simulink model "typeAsimctrl_NB_upgrade"  (R2017b)
settings: Solver=ode45  StartTime=0.0  StopTime=12.0  RelTol=1e-3  EnableMultiTasking=on
values from neighbouring files (symbols this model uses):
  gain_actIML = 2.1e-7*1.e+6*20/(2^16)/magIM(inddc)*gain_actIML    [TypeA_reconstruction.m]
  gain_actMNL = 5.1e-6*1.e+6*20/(2^16)/magMN(inddc)*gain_actMNL    [TypeA_reconstruction.m]
  gain_actTML = 1.7e-7*1.e+6*20/(2^16)/magTM(inddc)*gain_actTML    [TypeA_reconstruction.m]
  gainBFL = 0    [main.m]
  gainIPL = 0    [main.m]
  gainSCL = 1    [TypeA_reconstruction.m]
  gainSCT = 1    [TypeA_reconstruction.m]
  sys1 = sys1_exp    [check_exportvsmake.m]    (also in sumcon2mdlconst_typeA.m = sus.ss)
undefined symbols (not defined in the file or in its folder): cMat_BF, cMat_IM, cMat_MN, cMat_TM, Filt, gain_actBFGAS, gain_actBFL, gain_actBFP, gain_actBFR, gain_actBFT, gain_actBFV, gain_actBFY, gain_actF0GAS, gain_actF1GAS, gain_actF2GAS, gain_actF3GAS, gain_actIMP, gain_actIMR, gain_actIMT, gain_actIMV, gain_actIMY, gain_actIPL, gain_actIPT, gain_actIPY, gain_actMNP, gain_actMNR, gain_actMNT, gain_actMNV, gain_actMNY, gain_actTMP, gain_actTMY, gainBFP, gainBFR, gainBFT, gainBFV, gainBFY, gainBP, gainGASBF, gainGASF0, gainGASF1, gainGASF2, gainGASF3, gainIML, gainIMP, gainIMR, gainIMT, gainIMV, gainIMY, gainIPT, gainIPY, gainLOCK_IML, gainLOCK_IMP, gainLOCK_IMY, gainMNL, gainMNLOCK_L, gainMNLOCK_P, gainMNLOCK_Y, gainMNP, gainMNR, gainMNT ... (+22)
libraries: cstblocks x77, LiveParts x77
(part 1 of 3)
settings Model: Creator=kokioktm  LastModifiedBy=ayaka
settings DataIOCC: LimitDataPoints=on  SaveFormat=Array
settings OptimizationCC: LifeSpan=inf
settings DebuggingCC: SolverPrmCheckMsg=warning  SFUnexpectedBacktrackingDiag=warning  SFNoUnconditionalDefaultTransitionDiag=warning  SFExecutionAtInitializationDiag=none
settings HardwareCC: ProdBitPerPointer=32  ProdBitPerSizeT=32  ProdBitPerPtrDiffT=32  ProdLargestAtomicFloat=None  ProdIntDivRoundTo=Undefined  ProdEndianess=Unspecified  ProdWordSize=32  ProdHWDeviceType=32-bit Generic
settings ModelReferenceCC: PropagateSignalLabelsOutOfModel=off
settings CodeAppCC: StateflowObjectComments=on
settings GRTTargetCC: TargetLangStandard=C89/C90 (ANSI)  GeneratePreprocessorConditionals=Disable all
settings ConfigComp: CovMetricSettings=dw  CovHtmlReporting=on  CovSaveCumulativeToWorkspaceVar=on  CovSaveSingleToWorkspaceVar=on  CovExternalEMLEnable=off  CovSFcnEnable=off

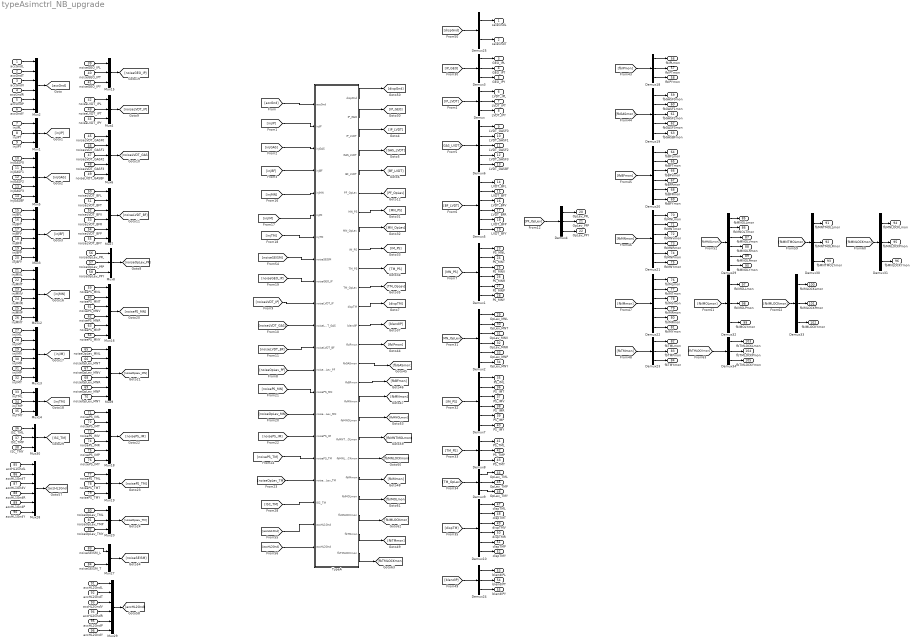
== system typeAsimctrl_NB_upgrade ==
  accGndL : Inport
  accGndT : Inport  Port=2
  accGndV : Inport  Port=3
  accGndR : Inport  Port=4
  accGndP : Inport  Port=5
  accGndY : Inport  Port=6
  injIPL : Inport  Port=7
  injIPT : Inport  Port=8
  injIPY : Inport  Port=9
  injGASF0 : Inport  Port=10
  injGASF1 : Inport  Port=11
  injGASF2 : Inport  Port=12
  injGASF3 : Inport  Port=13
  injGASBF : Inport  Port=14
  injBFL : Inport  Port=15
  injBFT : Inport  Port=16
  injBFV : Inport  Port=17
  injBFR : Inport  Port=18
  injBFP : Inport  Port=19
  injBFY : Inport  Port=20
  injMNL : Inport  Port=21
  injMNT : Inport  Port=22
  injMNV : Inport  Port=23
  injMNR : Inport  Port=24
  injMNP : Inport  Port=25
  injMNY : Inport  Port=26
  injIML : Inport  Port=27
  injIMT : Inport  Port=28
  injIMV : Inport  Port=29
  injIMR : Inport  Port=30
  injIMP : Inport  Port=31
  injIMY : Inport  Port=32
  injTML : Inport  Port=33
  injTMP : Inport  Port=34
  injTMY : Inport  Port=35
  ISC_TML : Inport  Port=36
  ISC_TMP : Inport  Port=37
  ISC_TMY : Inport  Port=38
  noiseGEO_IPL : Inport  Port=39
  noiseGEO_IPT : Inport  Port=40
  noiseGEO_IPY : Inport  Port=41
  noiseLVDT_IPL : Inport  Port=42
  noiseLVDT_IPT : Inport  Port=43
  noiseLVDT_IPY : Inport  Port=44
  noiseLVDT_GASF0 : Inport  Port=45
  noiseLVDT_GASF1 : Inport  Port=46
  noiseLVDT_GASF2 : Inport  Port=47
  noiseLVDT_GASF3 : Inport  Port=48
  noiseLVDT_GASBF : Inport  Port=49
  noiseLVDT_BFL : Inport  Port=50
  noiseLVDT_BFT : Inport  Port=51
  noiseLVDT_BFV : Inport  Port=52
  noiseLVDT_BFR : Inport  Port=53
  noiseLVDT_BFP : Inport  Port=54
  noiseLVDT_BFY : Inport  Port=55
  noiseOpLev_PFL : Inport  Port=56
  noiseOpLev_PFP : Inport  Port=57
  noiseOpLev_PFY : Inport  Port=58
  noisePS_MNL : Inport  Port=59
  noisePS_MNT : Inport  Port=60
  noisePS_MNV : Inport  Port=61
  noisePS_MNR : Inport  Port=62
  noisePS_MNP : Inport  Port=63
  noisePS_MNY : Inport  Port=64
  noiseOpLev_MNL : Inport  Port=65
  noiseOpLev_MNT : Inport  Port=66
  noiseOpLev_MNV : Inport  Port=67
  noiseOpLev_MNR : Inport  Port=68
  noiseOpLev_MNP : Inport  Port=69
  noiseOpLev_MNY : Inport  Port=70
  noisePS_IML : Inport  Port=71
  noisePS_IMT : Inport  Port=72
  noisePS_IMV : Inport  Port=73
  noisePS_IMR : Inport  Port=74
  noisePS_IMP : Inport  Port=75
  noisePS_IMY : Inport  Port=76
  noisePS_TML : Inport  Port=77
  noisePS_TMT : Inport  Port=78
  noisePS_TMY : Inport  Port=79
  noiseOpLev_TML : Inport  Port=80
  noiseOpLev_TMP : Inport  Port=81
  noiseOpLev_TMY : Inport  Port=82
  noiseSEISM_L : Inport  Port=83
  noiseSEISM_T : Inport  Port=84
  accHL1GndL : Inport  Port=85
  accHL1GndT : Inport  Port=86
  accHL1GndV : Inport  Port=87
  accHL1GndR : Inport  Port=88
  accHL1GndP : Inport  Port=89
  accHL1GndY : Inport  Port=90
  accHL2GndL : Inport  Port=91
  accHL2GndT : Inport  Port=92
  accHL2GndV : Inport  Port=93
  accHL2GndR : Inport  Port=94
  accHL2GndP : Inport  Port=95
  accHL2GndY : Inport  Port=96
  Demux{,3..4,8..9,18,23..24,30..34} (13 alike) : Demux  Outputs=3
  Demux{1..2,5,7,10,20..22,29} (9 alike) : Demux  Outputs=6
  Demux19 : Demux  Outputs=5
  Demux25 : Demux  Outputs=2
  Demux6 : Demux  Outputs=5
  Mux{1,4,8,14..15,19..20,30} (8 alike) : Mux  Inputs=3
  Mux{2..3,7,9,12..13,16,18,28..29} (10 alike) : Mux  Inputs=6
  Mux27 : Mux  Inputs=2
  Mux5 : Mux  Inputs=5
  Mux6 : Mux  Inputs=5
  TypeA : Subsystem
  seisGndL : Outport
  seisGndT : Outport  Port=2
  GEO_IPL : Outport  Port=3
  GEO_IPT : Outport  Port=4
  GEO_IPY : Outport  Port=5
  LVDT_IPL : Outport  Port=6
  LVDT_IPT : Outport  Port=7
  LVDT_IPY : Outport  Port=8
  LVDT_GASF0 : Outport  Port=9
  LVDT_GASF1 : Outport  Port=10
  LVDT_GASF2 : Outport  Port=11
  LVDT_GASF3 : Outport  Port=12
  LVDT_GASBF : Outport  Port=13
  LVDT_BFL : Outport  Port=14
  LVDT_BFT : Outport  Port=15
  LVDT_BFV : Outport  Port=16
  LVDT_BFR : Outport  Port=17
  LVDT_BFP : Outport  Port=18
  LVDT_BFY : Outport  Port=19
  OpLev_PFL : Outport  Port=20
  OpLev_PFP : Outport  Port=21
  OpLev_PFY : Outport  Port=22
  PS_MNL : Outport  Port=23
  PS_MNT : Outport  Port=24
  PS_MNV : Outport  Port=25
  PS_MNR : Outport  Port=26
  PS_MNP : Outport  Port=27
  PS_MNY : Outport  Port=28
  OpLev_MNL : Outport  Port=29
  OpLev_MNT : Outport  Port=30
  OpLev_MNV : Outport  Port=31
  OpLev_MNR : Outport  Port=32
  OpLev_MNP : Outport  Port=33
  OpLev_MNY : Outport  Port=34
  PS_IML : Outport  Port=35
  PS_IMT : Outport  Port=36
  PS_IMV : Outport  Port=37
  PS_IMR : Outport  Port=38
  PS_IMP : Outport  Port=39
  PS_IMY : Outport  Port=40
  PS_TML : Outport  Port=41
  PS_TMP : Outport  Port=42
  PS_TMY : Outport  Port=43
  OpLev_TML : Outport  Port=44
  OpLev_TMP : Outport  Port=45
  OpLev_TMY : Outport  Port=46
  dispTML : Outport  Port=47
  dispTMT : Outport  Port=48
  dispTMV : Outport  Port=49
  dispTMR : Outport  Port=50
  dispTMP : Outport  Port=51
  dispTMY : Outport  Port=52
  blendIPL : Outport  Port=53
  blendIPT : Outport  Port=54
  blendIPY : Outport  Port=55
  fbIPLmon : Outport  Port=56
  fbIPTmon : Outport  Port=57
  fbIPYmon : Outport  Port=58
  fbGASF0mon : Outport  Port=59
  fbGASF1mon : Outport  Port=60
  fbGASF2mon : Outport  Port=61
  fbGASF3mon : Outport  Port=62
  fbGASBFmon : Outport  Port=63
  fbBFLmon : Outport  Port=64
  fbBFTmon : Outport  Port=65
  fbBFVmon : Outport  Port=66
  fbBFRmon : Outport  Port=67
  fbBFPmon : Outport  Port=68
  fbBFYmon : Outport  Port=69
  fbMNLmon : Outport  Port=70
  fbMNTmon : Outport  Port=71
  fbMNVmon : Outport  Port=72
  fbMNRmon : Outport  Port=73
  fbMNPmon : Outport  Port=74
  fbMNYmon : Outport  Port=75
  fbIMLmon : Outport  Port=76
  fbIMTmon : Outport  Port=77
  fbIMVmon : Outport  Port=78
  fbIMRmon : Outport  Port=79
  fbIMPmon : Outport  Port=80
  fbIMYmon : Outport  Port=81
  fbTMLmon : Outport  Port=82
  fbTMPmon : Outport  Port=83
  fbTMYmon : Outport  Port=84
  fbMNOLLmon : Outport  Port=85
  fbMNOLTmon : Outport  Port=86
  fbMNOLVmon : Outport  Port=87
  fbMNOLRmon : Outport  Port=88
  fbMNOLPmon : Outport  Port=89
  fbMNOLYmon : Outport  Port=90
  fbMNTMOLLmon : Outport  Port=91
  fbMNTMOLPmon : Outport  Port=92
  fbMNTMOLYmon : Outport  Port=93
  fbMNLOCKLmon : Outport  Port=94
  fbMNLOCKPmon : Outport  Port=95
  fbMNLOCKYmon : Outport  Port=96
  fbIMOLLmon : Outport  Port=97
  fbIMOLPmon : Outport  Port=98
  fbIMOLYmon : Outport  Port=99
  fbIMLOCKLmon : Outport  Port=100
  fbIMLOCKPmon : Outport  Port=101
  fbIMLOCKYmon : Outport  Port=102
  fbTMLOCKLmon : Outport  Port=103
  fbTMLOCKPmon : Outport  Port=104
  fbTMLOCKYmon : Outport  Port=105
  wires:
  [accGnd] -> TypeA/1(accGnd)
  accGndT/1 -> Mux2/2
  accGndL/1 -> Mux2/1
  accGndV/1 -> Mux2/3
  accGndR/1 -> Mux2/4
  accGndP/1 -> Mux2/5
  accGndY/1 -> Mux2/6
  Mux2/1 -> [accGnd]
  injIPL/1 -> Mux1/1
  injIPT/1 -> Mux1/2
  injIPY/1 -> Mux1/3
  Mux1/1 -> [injIP]
  [injIP] -> TypeA/2(injIP)
  injGASF0/1 -> Mux5/1
  injGASF1/1 -> Mux5/2
  injGASF2/1 -> Mux5/3
  injGASF3/1 -> Mux5/4
  injGASBF/1 -> Mux5/5
  Mux5/1 -> [injGAS]
  [injGAS] -> TypeA/3(injGAS)
  injBFT/1 -> Mux3/2
  injBFL/1 -> Mux3/1
  injBFV/1 -> Mux3/3
  injBFR/1 -> Mux3/4
  injBFP/1 -> Mux3/5
  injBFY/1 -> Mux3/6
  Mux3/1 -> [injBF]
  [injBF] -> TypeA/4(injBF)
  TypeA/3(IP_LVDT) -> [IP_LVDT]
  TypeA/4(GAS_LVDT) -> [GAS_LVDT]
  TypeA/5(BF_LVDT) -> [BF_LVDT]
  TypeA/12(dispTM) -> [dispTM]
  [IP_LVDT] -> Demux/1
  Demux/1 -> LVDT_IPL/1
  Demux/2 -> LVDT_IPT/1
  Demux/3 -> LVDT_IPY/1
  [GAS_LVDT] -> Demux6/1
  Demux6/1 -> LVDT_GASF0/1
  Demux6/2 -> LVDT_GASF1/1
  Demux6/3 -> LVDT_GASF2/1
  Demux6/4 -> LVDT_GASF3/1
  Demux6/5 -> LVDT_GASBF/1
  [BF_LVDT] -> Demux5/1
  Demux5/1 -> LVDT_BFL/1
  Demux5/2 -> LVDT_BFT/1
  Demux5/3 -> LVDT_BFV/1
  Demux5/4 -> LVDT_BFR/1
  Demux5/5 -> LVDT_BFP/1
  Demux5/6 -> LVDT_BFY/1
  Demux1/1 -> PS_MNL/1
  Demux1/2 -> PS_MNT/1
  Demux1/3 -> PS_MNV/1
  Demux1/4 -> PS_MNR/1
  Demux1/5 -> PS_MNP/1
  Demux1/6 -> PS_MNY/1
  [MN_PS] -> Demux1/1
  noiseLVDT_IPL/1 -> Mux4/1
  noiseLVDT_IPT/1 -> Mux4/2
  noiseLVDT_IPY/1 -> Mux4/3
  Mux4/1 -> [noiseLVDT_IP]
  noiseLVDT_GASF0/1 -> Mux6/1
  noiseLVDT_GASF1/1 -> Mux6/2
  noiseLVDT_GASF2/1 -> Mux6/3
  noiseLVDT_GASF3/1 -> Mux6/4
  noiseLVDT_GASBF/1 -> Mux6/5
  Mux6/1 -> [noiseLVDT_GAS]
  noiseLVDT_BFT/1 -> Mux7/2
  noiseLVDT_BFL/1 -> Mux7/1
  noiseLVDT_BFV/1 -> Mux7/3
  noiseLVDT_BFR/1 -> Mux7/4
  noiseLVDT_BFP/1 -> Mux7/5
  noiseLVDT_BFY/1 -> Mux7/6
  Mux7/1 -> [noiseLVDT_BF]
  [noiseLVDT_IP] -> TypeA/10(noiseLVDT_IP)
  [noiseLVDT_GAS] -> TypeA/11(noiseLVDT_GAS)
  [noiseLVDT_BF] -> TypeA/12(noiseLVDT_BF)
  [injMN] -> TypeA/5(injMN)
  [injTM] -> TypeA/7(injTM)
  [injIM] -> TypeA/6(injIM)
  injMNT/1 -> Mux12/2
  injMNL/1 -> Mux12/1
  injMNV/1 -> Mux12/3
  injMNR/1 -> Mux12/4
  injMNP/1 -> Mux12/5
  injMNY/1 -> Mux12/6
  Mux12/1 -> [injMN]
  injIMT/1 -> Mux13/2
  injIML/1 -> Mux13/1
  injIMV/1 -> Mux13/3
  injIMR/1 -> Mux13/4
  injIMP/1 -> Mux13/5
  injIMY/1 -> Mux13/6
  Mux13/1 -> [injIM]
  injTML/1 -> Mux14/1
  injTMP/1 -> Mux14/2
  injTMY/1 -> Mux14/3
  Mux14/1 -> [injTM]
  noiseGEO_IPL/1 -> Mux15/1
  noiseGEO_IPT/1 -> Mux15/2
  noiseGEO_IPY/1 -> Mux15/3
  Mux15/1 -> [noiseGEO_IP]
  [noiseGEO_IP] -> TypeA/9(noiseGEO_IP)
  noisePS_MNT/1 -> Mux16/2
  noisePS_MNL/1 -> Mux16/1
  noisePS_MNV/1 -> Mux16/3
  noisePS_MNR/1 -> Mux16/4
  noisePS_MNP/1 -> Mux16/5
  noisePS_MNY/1 -> Mux16/6
  Mux16/1 -> [noisePS_MN]
  noiseOpLev_MNR/1 -> Mux9/4
  noiseOpLev_MNP/1 -> Mux9/5
  Mux9/1 -> [noiseOpLev_MN]
  noiseOpLev_MNY/1 -> Mux9/6
  noisePS_IMT/1 -> Mux18/2
  noisePS_IML/1 -> Mux18/1
  noisePS_IMV/1 -> Mux18/3
  noisePS_IMR/1 -> Mux18/4
  noisePS_IMP/1 -> Mux18/5
  noisePS_IMY/1 -> Mux18/6
  Mux18/1 -> [noisePS_IM]
  noisePS_TML/1 -> Mux19/1
  noisePS_TMT/1 -> Mux19/2
  Mux19/1 -> [noisePS_TM]
  noisePS_TMY/1 -> Mux19/3
  noiseOpLev_TMP/1 -> Mux20/2
  noiseOpLev_TMY/1 -> Mux20/3
  Mux20/1 -> [noiseOpLev_TM]
  [noisePS_MN] -> TypeA/14(noisePS_MN)
  [noisePS_IM] -> TypeA/16(noisePS_IM)
  [noiseOpLev_MN] -> TypeA/15(noiseOpLev_MN)
  [noisePS_TM] -> TypeA/17(noisePS_TM)
  [noiseOpLev_TM] -> TypeA/18(noiseOpLev_TM)
  [ISC_TM] -> TypeA/19(ISC_TM)
  [IP_GEO] -> Demux3/1
  Demux3/1 -> GEO_IPL/1
  Demux3/2 -> GEO_IPT/1
  Demux3/3 -> GEO_IPY/1
  TypeA/2(IP_GEO) -> [IP_GEO]
  TypeA/9(IM_PS) -> [IM_PS]
  TypeA/10(TM_PS) -> [TM_PS]
  TypeA/8(MN_OpLev) -> [MN_OpLev]
  TypeA/7(MN_PS) -> [MN_PS]
  TypeA/11(TM_OpLev) -> [TM_OpLev]
  TypeA/15(fbGASmon) -> [fbGASmon]
  TypeA/14(fbIPmon) -> [fbIPmon]
  TypeA/24(fbTMmon) -> [fbTMmon]
  TypeA/17(fbMNmon) -> [fbMNmon]
  TypeA/13(blendIP) -> [blendIP]
  TypeA/21(fbIMmon) -> [fbIMmon]
  TypeA/16(fbBFmon) -> [fbBFmon]
  [MN_OpLev] -> Demux2/1
  Demux2/5 -> OpLev_MNP/1
  Demux2/6 -> OpLev_MNY/1
  Demux2/4 -> OpLev_MNR/1
  Demux7/1 -> PS_IML/1
  Demux7/2 -> PS_IMT/1
  Demux7/3 -> PS_IMV/1
  Demux7/4 -> PS_IMR/1
  Demux7/5 -> PS_IMP/1
  Demux7/6 -> PS_IMY/1
  [IM_PS] -> Demux7/1
  Demux8/1 -> PS_TML/1
  [TM_PS] -> Demux8/1
  Demux8/2 -> PS_TMP/1
  Demux8/3 -> PS_TMY/1
  [TM_OpLev] -> Demux9/1
  Demux10/1 -> dispTML/1
  Demux10/2 -> dispTMT/1
  Demux10/3 -> dispTMV/1
  Demux10/4 -> dispTMR/1
  Demux10/5 -> dispTMP/1
  Demux10/6 -> dispTMY/1
  [dispTM] -> Demux10/1
  [fbIPmon] -> Demux18/1
  Demux18/1 -> fbIPLmon/1
  Demux18/2 -> fbIPTmon/1
  Demux18/3 -> fbIPYmon/1
  [fbGASmon] -> Demux19/1
  Demux19/1 -> fbGASF0mon/1
  Demux19/2 -> fbGASF1mon/1
  Demux19/3 -> fbGASF2mon/1
  Demux19/4 -> fbGASF3mon/1
  Demux19/5 -> fbGASBFmon/1
  [fbBFmon] -> Demux20/1
  Demux20/1 -> fbBFLmon/1
  Demux20/2 -> fbBFTmon/1
  Demux20/3 -> fbBFVmon/1
  Demux20/4 -> fbBFRmon/1
  Demux20/5 -> fbBFPmon/1
  Demux20/6 -> fbBFYmon/1
  [fbMNmon] -> Demux21/1
  Demux21/1 -> fbMNLmon/1
  Demux21/2 -> fbMNTmon/1
  Demux21/3 -> fbMNVmon/1
  Demux21/4 -> fbMNRmon/1
  Demux21/5 -> fbMNPmon/1
  Demux21/6 -> fbMNYmon/1
  [fbIMmon] -> Demux22/1
  Demux22/1 -> fbIMLmon/1
  Demux22/2 -> fbIMTmon/1
  Demux22/3 -> fbIMVmon/1
  Demux22/4 -> fbIMRmon/1
  Demux22/5 -> fbIMPmon/1
  Demux22/6 -> fbIMYmon/1
  [fbTMmon] -> Demux23/1
  Demux23/2 -> fbTMPmon/1
  Demux23/3 -> fbTMYmon/1
  Demux23/1 -> fbTMLmon/1
  Demux24/1 -> blendIPL/1
  [blendIP] -> Demux24/1
  Demux24/2 -> blendIPT/1
  Demux24/3 -> blendIPY/1
  [dispGnd] -> Demux25/1
  Demux25/1 -> seisGndL/1
  Demux25/2 -> seisGndT/1
  TypeA/1(dispGnd) -> [dispGnd]
  noiseOpLev_TML/1 -> Mux20/1
  [noiseSEISM] -> TypeA/8(noiseSEISM)
  noiseSEISM_T/1 -> Mux27/2
  Mux27/1 -> [noiseSEISM]
  noiseSEISM_L/1 -> Mux27/1
  [accHL1Gnd] -> TypeA/20(accHL1Gnd)
  [accHL2Gnd] -> TypeA/21(accHL2Gnd)
  accHL1GndT/1 -> Mux28/2
  accHL1GndL/1 -> Mux28/1
  accHL1GndV/1 -> Mux28/3
  accHL1GndR/1 -> Mux28/4
  accHL1GndP/1 -> Mux28/5
  accHL1GndY/1 -> Mux28/6
  Mux28/1 -> [accHL1Gnd]
  accHL2GndT/1 -> Mux29/2
  accHL2GndL/1 -> Mux29/1
  accHL2GndV/1 -> Mux29/3
  accHL2GndR/1 -> Mux29/4
  accHL2GndP/1 -> Mux29/5
  accHL2GndY/1 -> Mux29/6
  Mux29/1 -> [accHL2Gnd]
  TypeA/20(fbMNLOCKmon) -> [fbMNLOCKmon]
  TypeA/19(fbMNTMOLmon) -> [fbMNTMOLmon]
  TypeA/18(fbMNOLmon) -> [fbMNOLmon]
  TypeA/22(fbIMOLmon) -> [fbIMOLmon]
  TypeA/23(fbIMLOCKmon) -> [fbIMLOCKmon]
  TypeA/25(fbTMLOCKmon) -> [fbTMLOCKmon]
  [fbMNOLmon] -> Demux29/1
  [fbMNTMOLmon] -> Demux30/1
  Demux30/1 -> fbMNTMOLLmon/1
  Demux30/2 -> fbMNTMOLPmon/1
  Demux30/3 -> fbMNTMOLYmon/1
  [fbMNLOCKmon] -> Demux31/1
  Demux31/1 -> fbMNLOCKLmon/1
  Demux31/2 -> fbMNLOCKPmon/1
  Demux31/3 -> fbMNLOCKYmon/1
  [fbIMOLmon] -> Demux32/1
  Demux32/1 -> fbIMOLLmon/1
  Demux32/2 -> fbIMOLPmon/1
  Demux32/3 -> fbIMOLYmon/1
  [fbIMLOCKmon] -> Demux33/1
  Demux33/1 -> fbIMLOCKLmon/1
  Demux33/2 -> fbIMLOCKPmon/1
  Demux33/3 -> fbIMLOCKYmon/1
  [fbTMLOCKmon] -> Demux34/1
  Demux34/2 -> fbTMLOCKPmon/1
  Demux34/3 -> fbTMLOCKYmon/1
  Demux34/1 -> fbTMLOCKLmon/1
  Mux30/1 -> [ISC_TM]
  ISC_TML/1 -> Mux30/1
  ISC_TMP/1 -> Mux30/2
  ISC_TMY/1 -> Mux30/3
  [noiseOpLev_PF] -> TypeA/13(noiseOpLev_PF)
  noiseOpLev_PFL/1 -> Mux8/1
  noiseOpLev_PFY/1 -> Mux8/3
  Mux8/1 -> [noiseOpLev_PF]
  noiseOpLev_PFP/1 -> Mux8/2
  noiseOpLev_MNT/1 -> Mux9/2
  noiseOpLev_MNV/1 -> Mux9/3
  noiseOpLev_MNL/1 -> Mux9/1
  Demux2/3 -> OpLev_MNV/1
  Demux2/2 -> OpLev_MNT/1
  Demux2/1 -> OpLev_MNL/1
  TypeA/6(PF_OpLev) -> [PF_OpLev]
  Demux9/1 -> OpLev_TML/1
  Demux9/2 -> OpLev_TMP/1
  Demux9/3 -> OpLev_TMY/1
  Demux4/3 -> OpLev_PFY/1
  Demux4/1 -> OpLev_PFL/1
  Demux4/2 -> OpLev_PFP/1
  [PF_OpLev] -> Demux4/1
  Demux29/6 -> fbMNOLYmon/1
  Demux29/5 -> fbMNOLPmon/1
  Demux29/1 -> fbMNOLLmon/1
  Demux29/2 -> fbMNOLTmon/1
  Demux29/3 -> fbMNOLVmon/1
  Demux29/4 -> fbMNOLRmon/1

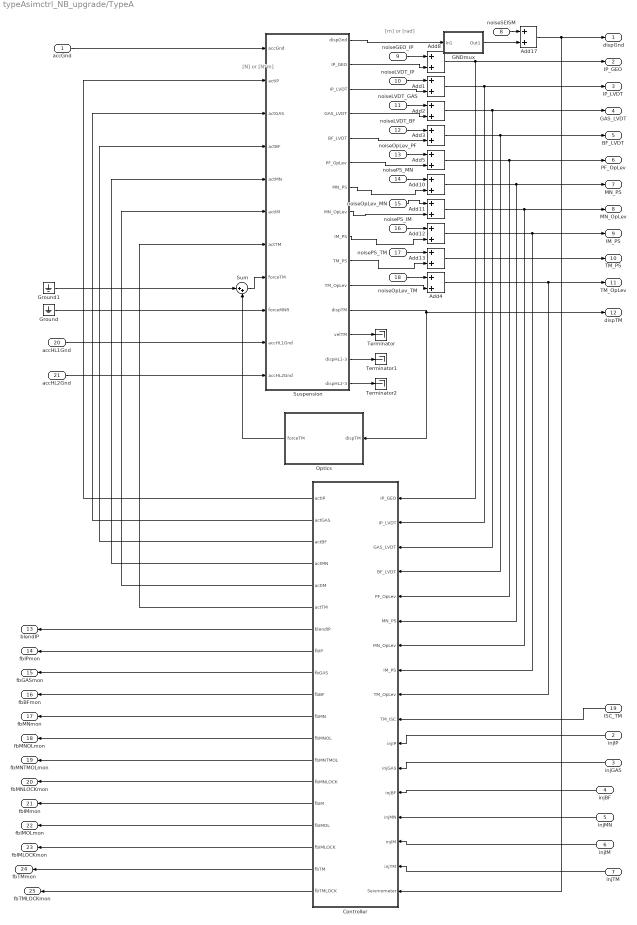
== system typeAsimctrl_NB_upgrade/TypeA ==
  note: [N] or [N*m]
  note: [m] or [rad]
  accGnd : Inport
  injIP : Inport  Port=2
  injGAS : Inport  Port=3
  injBF : Inport  Port=4
  injMN : Inport  Port=5
  injIM : Inport  Port=6
  injTM : Inport  Port=7
  noiseSEISM : Inport  Port=8
  noiseGEO_IP : Inport  Port=9
  noiseLVDT_IP : Inport  Port=10
  noiseLVDT_GAS : Inport  Port=11
  noiseLVDT_BF : Inport  Port=12
  noiseOpLev_PF : Inport  Port=13
  noisePS_MN : Inport  Port=14
  noiseOpLev_MN : Inport  Port=15
  noisePS_IM : Inport  Port=16
  noisePS_TM : Inport  Port=17
  noiseOpLev_TM : Inport  Port=18
  ISC_TM : Inport  Port=19
  accHL1Gnd : Inport  Port=20
  accHL2Gnd : Inport  Port=21
  Add{1..5,8,10..13,17} (11 alike) : Sum
  Controller : Subsystem
  GNDmux : Subsystem
  Ground : Ground
  Ground1 : Ground
  Optics : Subsystem
  Sum : Sum  Inputs=|++
  Suspension : Subsystem
  Terminator : Terminator
  Terminator1 : Terminator
  Terminator2 : Terminator
  dispGnd : Outport
  IP_GEO : Outport  Port=2
  IP_LVDT : Outport  Port=3
  GAS_LVDT : Outport  Port=4
  BF_LVDT : Outport  Port=5
  PF_OpLev : Outport  Port=6
  MN_PS : Outport  Port=7
  MN_OpLev : Outport  Port=8
  IM_PS : Outport  Port=9
  TM_PS : Outport  Port=10
  TM_OpLev : Outport  Port=11
  dispTM : Outport  Port=12
  blendIP : Outport  Port=13
  fbIPmon : Outport  Port=14
  fbGASmon : Outport  Port=15
  fbBFmon : Outport  Port=16
  fbMNmon : Outport  Port=17
  fbMNOLmon : Outport  Port=18
  fbMNTMOLmon : Outport  Port=19
  fbMNLOCKmon : Outport  Port=20
  fbIMmon : Outport  Port=21
  fbIMOLmon : Outport  Port=22
  fbIMLOCKmon : Outport  Port=23
  fbTMmon : Outport  Port=24
  fbTMLOCKmon : Outport  Port=25
  wires:
  Add1/1 -> IP_LVDT/1, Controller/2(IP_LVDT)
  Add3/1 -> Controller/4(BF_LVDT), BF_LVDT/1
  Add2/1 -> GAS_LVDT/1, Controller/3(GAS_LVDT)
  Controller/1(actIP) -> Suspension/2(actIP)
  Controller/3(actBF) -> Suspension/4(actBF)
  Add4/1 -> Controller/9(TM_OpLev), TM_OpLev/1
  accGnd/1 -> Suspension/1(accGnd)
  Controller/2(actGAS) -> Suspension/3(actGAS)
  injGAS/1 -> Controller/12(injGAS)
  injIP/1 -> Controller/11(injIP)
  injBF/1 -> Controller/13(injBF)
  Controller/10(fbBF) -> fbBFmon/1
  Controller/8(fbIP) -> fbIPmon/1
  Controller/9(fbGAS) -> fbGASmon/1
  Suspension/3(IP_LVDT) -> Add1/2
  Suspension/4(GAS_LVDT) -> Add2/2
  Suspension/5(BF_LVDT) -> Add3/2
  Suspension/11(TM_OpLev) -> Add4/2
  noiseLVDT_IP/1 -> Add1/1
  noiseLVDT_GAS/1 -> Add2/1
  noiseLVDT_BF/1 -> Add3/1
  noiseOpLev_TM/1 -> Add4/1
  Add8/1 -> Controller/1(IP_GEO), IP_GEO/1
  noiseGEO_IP/1 -> Add8/1
  Suspension/2(IP_GEO) -> Add8/2
  noisePS_MN/1 -> Add10/1
  Add10/1 -> Controller/6(MN_PS), MN_PS/1
  noiseOpLev_MN/1 -> Add11/1
  Add11/1 -> Controller/7(MN_OpLev), MN_OpLev/1
  noisePS_IM/1 -> Add12/1
  Add12/1 -> Controller/8(IM_PS), IM_PS/1
  Suspension/8(MN_OpLev) -> Add11/2
  Suspension/7(MN_PS) -> Add10/2
  Suspension/9(IM_PS) -> Add12/2
  noisePS_TM/1 -> Add13/1
  Add13/1 -> TM_PS/1
  Suspension/10(TM_PS) -> Add13/2
  injMN/1 -> Controller/14(injMN)
  injTM/1 -> Controller/16(injTM)
  injIM/1 -> Controller/15(injIM)
  Controller/4(actMN) -> Suspension/5(actMN)
  Controller/5(actIM) -> Suspension/6(actIM)
  Controller/6(actTM) -> Suspension/7(actTM)
  Controller/7(blendIP) -> blendIP/1
  Controller/18(fbTM) -> fbTMmon/1
  Controller/11(fbMN) -> fbMNmon/1
  Controller/15(fbIM) -> fbIMmon/1
  Ground/1 -> Suspension/9(forceMNR)
  noiseSEISM/1 -> Add17/1
  Add17/1 -> Controller/17(Seismometer), dispGnd/1
  Suspension/12(dispTM) -> Optics/1(dispTM), dispTM/1
  Optics/1(forceTM) -> Sum/2
  Ground1/1 -> Sum/1
  Sum/1 -> Suspension/8(forceTM)
  Suspension/1(dispGnd) -> GNDmux/1(In1)
  GNDmux/1(Out1) -> Add17/2
  accHL1Gnd/1 -> Suspension/10(accHL1Gnd)
  accHL2Gnd/1 -> Suspension/11(accHL2Gnd)
  Controller/12(fbMNOL) -> fbMNOLmon/1
  Controller/13(fbMNTMOL) -> fbMNTMOLmon/1
  Controller/14(fbMNLOCK) -> fbMNLOCKmon/1
  Controller/16(fbIMOL) -> fbIMOLmon/1
  Controller/17(fbIMLOCK) -> fbIMLOCKmon/1
  Controller/19(fbTMLOCK) -> fbTMLOCKmon/1
  Suspension/13(velTM) -> Terminator/1
  Suspension/14(dispHL1-3) -> Terminator1/1
  Suspension/15(dispHL2-3) -> Terminator2/1
  Suspension/6(PF_OpLev) -> Add5/2
  noiseOpLev_PF/1 -> Add5/1
  Add5/1 -> Controller/5(PF_OpLev), PF_OpLev/1
  ISC_TM/1 -> Controller/10(TM_ISC)

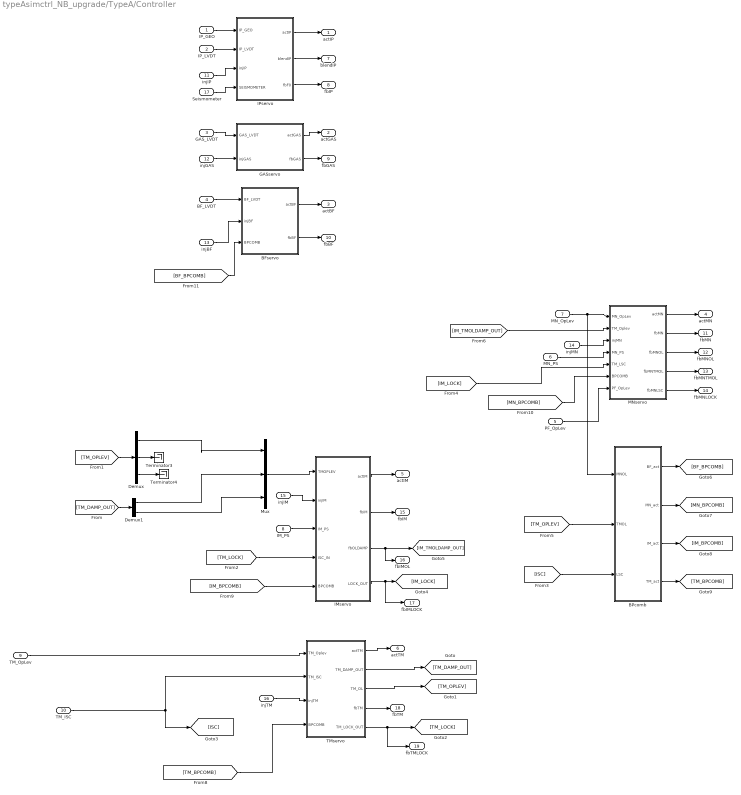
== system typeAsimctrl_NB_upgrade/TypeA/Controller ==
  IP_GEO : Inport
  IP_LVDT : Inport  Port=2
  GAS_LVDT : Inport  Port=3
  BF_LVDT : Inport  Port=4
  PF_OpLev : Inport  Port=5
  MN_PS : Inport  Port=6
  MN_OpLev : Inport  Port=7
  IM_PS : Inport  Port=8
  TM_OpLev : Inport  Port=9
  TM_ISC : Inport  Port=10
  injIP : Inport  Port=11
  injGAS : Inport  Port=12
  injBF : Inport  Port=13
  injMN : Inport  Port=14
  injIM : Inport  Port=15
  injTM : Inport  Port=16
  Seismometer : Inport  Port=17
  BFservo : Subsystem
  BPcomb : Subsystem
  Demux : Demux  Outputs=3
  Demux1 : Demux  Outputs=2
  GASservo : Subsystem
  IMservo : Subsystem
  IPservo : Subsystem
  MNservo : Subsystem
  Mux : Mux  Inputs=3
  TMservo : Subsystem
  Terminator3 : Terminator
  Terminator4 : Terminator
  actIP : Outport
  actGAS : Outport  Port=2
  actBF : Outport  Port=3
  actMN : Outport  Port=4
  actIM : Outport  Port=5
  actTM : Outport  Port=6
  blendIP : Outport  Port=7
  fbIP : Outport  Port=8
  fbGAS : Outport  Port=9
  fbBF : Outport  Port=10
  fbMN : Outport  Port=11
  fbMNOL : Outport  Port=12
  fbMNTMOL : Outport  Port=13
  fbMNLOCK : Outport  Port=14
  fbIM : Outport  Port=15
  fbIMOL : Outport  Port=16
  fbIMLOCK : Outport  Port=17
  fbTM : Outport  Port=18
  fbTMLOCK : Outport  Port=19
  wires:
  IP_LVDT/1 -> IPservo/2(IP_LVDT)
  injIP/1 -> IPservo/3(injIP)
  IPservo/3(fbF0) -> fbIP/1
  IPservo/1(actIP) -> actIP/1
  GASservo/1(actGAS) -> actGAS/1
  GASservo/2(fbGAS) -> fbGAS/1
  GAS_LVDT/1 -> GASservo/1(GAS_LVDT)
  injGAS/1 -> GASservo/2(injGAS)
  BF_LVDT/1 -> BFservo/1(BF_LVDT)
  injBF/1 -> BFservo/2(injBF)
  BFservo/1(actBF) -> actBF/1
  BFservo/2(fbBF) -> fbBF/1
  IP_GEO/1 -> IPservo/1(IP_GEO)
  IPservo/2(blendIP) -> blendIP/1
  TM_OpLev/1 -> TMservo/1(TM_Oplev)
  injTM/1 -> TMservo/3(injTM)
  MN_OpLev/1 -> BPcomb/1(MNOL), MNservo/1(MN_OpLev)
  injMN/1 -> MNservo/3(injMN)
  injIM/1 -> IMservo/2(injIM)
  TMservo/1(actTM) -> actTM/1
  TMservo/4(fbTM) -> fbTM/1
  IMservo/2(fbIM) -> fbIM/1
  IMservo/1(actIM) -> actIM/1
  MNservo/2(fbMN) -> fbMN/1
  MNservo/1(actMN) -> actMN/1
  MN_PS/1 -> MNservo/4(MN_PS)
  IM_PS/1 -> IMservo/3(IM_PS)
  TMservo/2(TM_DAMP_OUT) -> [TM_DAMP_OUT]
  [TM_OPLEV] -> Demux/1
  Demux/1 -> Mux/1
  Mux/1 -> IMservo/1(TMOPLEV)
  [TM_DAMP_OUT] -> Demux1/1
  TMservo/3(TM_OL) -> [TM_OPLEV]
  [TM_LOCK] -> IMservo/4(ISC_IN)
  IMservo/4(LOCK_OUT) -> fbIMLOCK/1, [IM_LOCK]
  [IM_LOCK] -> MNservo/5(TM_LSC)
  [IM_TMOLDAMP_OUT] -> MNservo/2(TM_Oplev)
  IMservo/3(fbOLDAMP) -> fbIMOL/1, [IM_TMOLDAMP_OUT]
  Seismometer/1 -> IPservo/4(SEISMOMETER)
  Demux1/1 -> Mux/2
  Demux1/2 -> Mux/3
  Demux/2 -> Terminator3/1
  Demux/3 -> Terminator4/1
  [ISC] -> BPcomb/3(LSC)
  [TM_OPLEV] -> BPcomb/2(TMOL)
  BPcomb/4(TM_act) -> [TM_BPCOMB]
  BPcomb/3(IM_act) -> [IM_BPCOMB]
  BPcomb/2(MN_act) -> [MN_BPCOMB]
  BPcomb/1(BF_act) -> [BF_BPCOMB]
  [TM_BPCOMB] -> TMservo/4(BPCOMB)
  [IM_BPCOMB] -> IMservo/5(BPCOMB)
  [MN_BPCOMB] -> MNservo/6(BPCOMB)
  [BF_BPCOMB] -> BFservo/3(BPCOMB)
  TMservo/5(TM_LOCK_OUT) -> fbTMLOCK/1, [TM_LOCK]
  MNservo/5(fbMNLSC) -> fbMNLOCK/1
  MNservo/3(fbMNOL) -> fbMNOL/1
  MNservo/4(fbMNTMOL) -> fbMNTMOL/1
  TM_ISC/1 -> [ISC], TMservo/2(TM_ISC)
  PF_OpLev/1 -> MNservo/7(PF_OpLev)

== system typeAsimctrl_NB_upgrade/TypeA/GNDmux ==
  In1 : Inport
  Demux : Demux
  Mux : Mux  Inputs=2
  Terminator : Terminator
  Terminator1 : Terminator
  Out1 : Outport
  wires:
  Mux/1 -> Out1/1
  Demux/4 -> Terminator/1  "Y"
  Demux/1 -> Mux/1  "L"
  Demux/3 -> Terminator1/1  "V"
  In1/1 -> Demux/1
  Demux/2 -> Mux/2  "T"

== system typeAsimctrl_NB_upgrade/TypeA/Optics ==
  dispTM : Inport
  Demux : Demux  Outputs=6
  Ground : Ground
  Kopt_angle : Gain  Gain=Kopt_angle
  Kopt_angle1 : Gain  Gain=Kopt_angle
  Kopt_len : Gain  Gain=Kopt_len
  Mux : Mux  Inputs=6
  Terminator1 : Terminator
  Terminator2 : Terminator
  Terminator3 : Terminator
  forceTM : Outport
  wires:
  dispTM/1 -> Demux/1
  Demux/6 -> Kopt_angle1/1
  Kopt_angle1/1 -> Mux/6
  Demux/5 -> Kopt_angle/1
  Kopt_angle/1 -> Mux/5
  Demux/2 -> Terminator1/1
  Demux/3 -> Terminator2/1
  Demux/4 -> Terminator3/1
  Mux/1 -> forceTM/1
  Demux/1 -> Kopt_len/1
  Kopt_len/1 -> Mux/1
  Ground/1 -> Mux/4, Mux/3, Mux/2

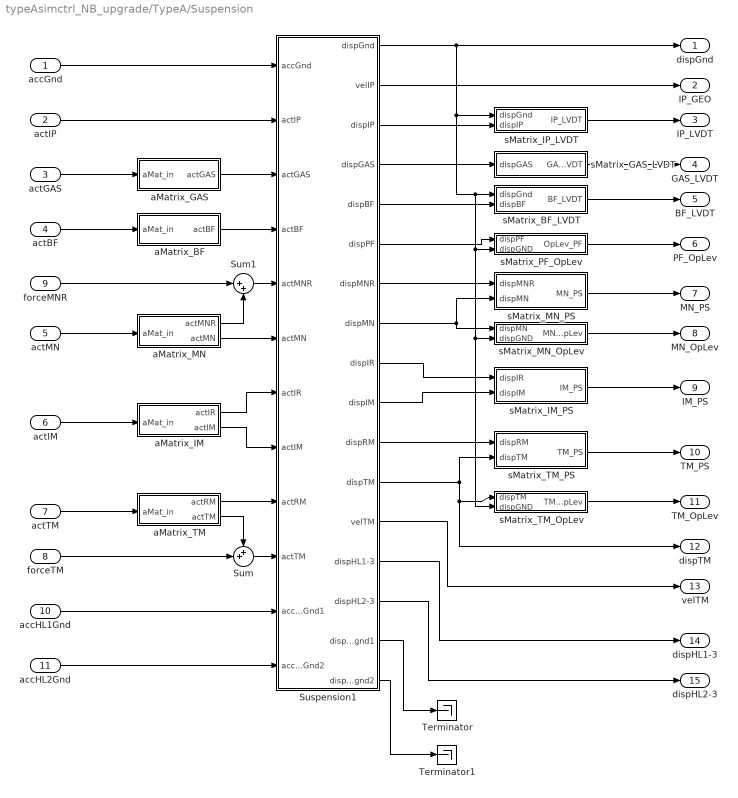
== system typeAsimctrl_NB_upgrade/TypeA/Suspension ==
  accGnd : Inport
  actIP : Inport  Port=2
  actGAS : Inport  Port=3
  actBF : Inport  Port=4
  actMN : Inport  Port=5
  actIM : Inport  Port=6
  actTM : Inport  Port=7
  forceTM : Inport  Port=8
  forceMNR : Inport  Port=9
  accHL1Gnd : Inport  Port=10
  accHL2Gnd : Inport  Port=11
  Sum : Sum  Inputs=++|
  Sum1 : Sum  Inputs=|++
  Suspension1 : Subsystem
  Terminator : Terminator
  Terminator1 : Terminator
  aMatrix_BF : Subsystem
  aMatrix_GAS : Subsystem
  aMatrix_IM : Subsystem
  aMatrix_MN : Subsystem
  aMatrix_TM : Subsystem
  sMatrix_BF_LVDT : Subsystem
  sMatrix_GAS_LVDT : Subsystem
  sMatrix_IM_PS : Subsystem
  sMatrix_IP_LVDT : Subsystem
  sMatrix_MN_OpLev : Subsystem
  sMatrix_MN_PS : Subsystem
  sMatrix_PF_OpLev : Subsystem
  sMatrix_TM_OpLev : Subsystem
  sMatrix_TM_PS : Subsystem
  dispGnd : Outport
  IP_GEO : Outport  Port=2
  IP_LVDT : Outport  Port=3
  GAS_LVDT : Outport  Port=4
  BF_LVDT : Outport  Port=5
  PF_OpLev : Outport  Port=6
  MN_PS : Outport  Port=7
  MN_OpLev : Outport  Port=8
  IM_PS : Outport  Port=9
  TM_PS : Outport  Port=10
  TM_OpLev : Outport  Port=11
  dispTM : Outport  Port=12
  velTM : Outport  Port=13
  dispHL1-3 : Outport  Port=14
  dispHL2-3 : Outport  Port=15
  wires:
  Suspension1/1(dispGnd) -> dispGnd/1, sMatrix_PF_OpLev/2(dispGND), sMatrix_MN_OpLev/2(dispGND), sMatrix_TM_OpLev/2(dispGND), sMatrix_BF_LVDT/1(dispGnd), sMatrix_IP_LVDT/1(dispGnd)
  Suspension1/3(dispIP) -> sMatrix_IP_LVDT/2(dispIP)
  Suspension1/4(dispGAS) -> sMatrix_GAS_LVDT/1(dispGAS)
  Suspension1/5(dispBF) -> sMatrix_BF_LVDT/2(dispBF)
  sMatrix_IP_LVDT/1(IP_LVDT) -> IP_LVDT/1
  sMatrix_GAS_LVDT/1(GAS_LVDT) -> GAS_LVDT/1
  sMatrix_BF_LVDT/1(BF_LVDT) -> BF_LVDT/1
  Suspension1/12(dispTM) -> dispTM/1, sMatrix_TM_OpLev/1(dispTM), sMatrix_TM_PS/2(dispTM)
  accGnd/1 -> Suspension1/1(accGnd)
  actIP/1 -> Suspension1/2(actIP)
  actGAS/1 -> aMatrix_GAS/1(aMat_in)
  actBF/1 -> aMatrix_BF/1(aMat_in)
  sMatrix_TM_OpLev/1(TM_OpLev) -> TM_OpLev/1
  aMatrix_GAS/1(actGAS) -> Suspension1/3(actGAS)
  aMatrix_BF/1(actBF) -> Suspension1/4(actBF)
  Suspension1/6(dispPF) -> sMatrix_PF_OpLev/1(dispPF)
  sMatrix_PF_OpLev/1(OpLev_PF) -> PF_OpLev/1
  Suspension1/7(dispMNR) -> sMatrix_MN_PS/1(dispMNR)
  Suspension1/8(dispMN) -> sMatrix_MN_PS/2(dispMN), sMatrix_MN_OpLev/1(dispMN)
  sMatrix_MN_PS/1(MN_PS) -> MN_PS/1
  sMatrix_MN_OpLev/1(MN_OpLev) -> MN_OpLev/1
  Suspension1/9(dispIR) -> sMatrix_IM_PS/1(dispIR)
  Suspension1/10(dispIM) -> sMatrix_IM_PS/2(dispIM)
  sMatrix_IM_PS/1(IM_PS) -> IM_PS/1
  Suspension1/11(dispRM) -> sMatrix_TM_PS/1(dispRM)
  sMatrix_TM_PS/1(TM_PS) -> TM_PS/1
  Suspension1/13(velTM) -> velTM/1
  aMatrix_MN/1(actMNR) -> Sum1/2
  aMatrix_MN/2(actMN) -> Suspension1/6(actMN)
  actMN/1 -> aMatrix_MN/1(aMat_in)
  actIM/1 -> aMatrix_IM/1(aMat_in)
  aMatrix_IM/1(actIR) -> Suspension1/7(actIR)
  aMatrix_IM/2(actIM) -> Suspension1/8(actIM)
  actTM/1 -> aMatrix_TM/1(aMat_in)
  aMatrix_TM/1(actRM) -> Suspension1/9(actRM)
  Sum/1 -> Suspension1/10(actTM)
  aMatrix_TM/2(actTM) -> Sum/1
  forceTM/1 -> Sum/2
  Suspension1/2(velIP) -> IP_GEO/1
  Sum1/1 -> Suspension1/5(actMNR)
  forceMNR/1 -> Sum1/1
  accHL1Gnd/1 -> Suspension1/11(accHLGnd1)
  accHL2Gnd/1 -> Suspension1/12(accHLGnd2)
  Suspension1/14(dispHL1-3) -> dispHL1-3/1
  Suspension1/15(dispHL2-3) -> dispHL2-3/1
  Suspension1/16(dispHLgnd1) -> Terminator/1
  Suspension1/17(dispHLgnd2) -> Terminator1/1

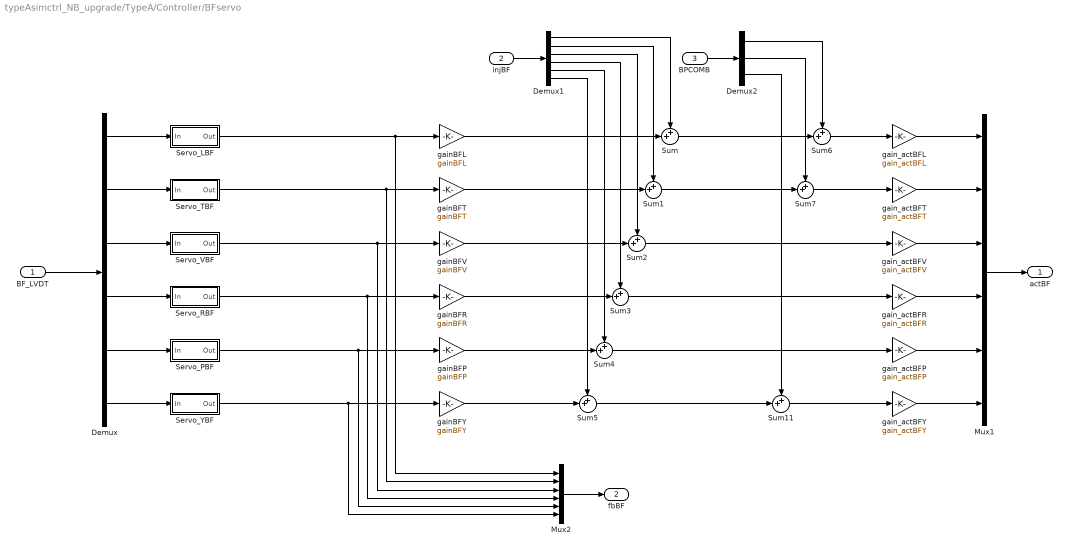
== system typeAsimctrl_NB_upgrade/TypeA/Controller/BFservo ==
  BF_LVDT : Inport
  injBF : Inport  Port=2
  BPCOMB : Inport  Port=3
  Demux : Demux  Outputs=6
  Demux1 : Demux  Outputs=6
  Demux2 : Demux  Outputs=3
  Mux1 : Mux  Inputs=6
  Mux2 : Mux  Inputs=6
  Servo_LBF : Subsystem
  Servo_PBF : Subsystem
  Servo_RBF : Subsystem
  Servo_TBF : Subsystem
  Servo_VBF : Subsystem
  Servo_YBF : Subsystem
  Sum{,1..7,11} (9 alike) : Sum  Inputs=++|
  gainBFL : Gain  Gain=gainBFL
  gainBFP : Gain  Gain=gainBFP
  gainBFR : Gain  Gain=gainBFR
  gainBFT : Gain  Gain=gainBFT
  gainBFV : Gain  Gain=gainBFV
  gainBFY : Gain  Gain=gainBFY
  gain_actBFL : Gain  Gain=gain_actBFL
  gain_actBFP : Gain  Gain=gain_actBFP
  gain_actBFR : Gain  Gain=gain_actBFR
  gain_actBFT : Gain  Gain=gain_actBFT
  gain_actBFV : Gain  Gain=gain_actBFV
  gain_actBFY : Gain  Gain=gain_actBFY
  actBF : Outport
  fbBF : Outport  Port=2
  wires:
  BF_LVDT/1 -> Demux/1
  Demux/1 -> Servo_LBF/1(In)
  Demux/2 -> Servo_TBF/1(In)
  Demux/3 -> Servo_VBF/1(In)
  Servo_LBF/1(Out) -> gainBFL/1, Mux2/1
  Servo_TBF/1(Out) -> gainBFT/1, Mux2/2
  Servo_VBF/1(Out) -> gainBFV/1, Mux2/3
  injBF/1 -> Demux1/1
  Sum2/1 -> gain_actBFV/1
  Mux1/1 -> actBF/1
  Mux2/1 -> fbBF/1
  Demux1/3 -> Sum2/1
  Demux1/2 -> Sum1/1
  Demux1/1 -> Sum/1
  Servo_RBF/1(Out) -> gainBFR/1, Mux2/4
  Servo_PBF/1(Out) -> gainBFP/1, Mux2/5
  Demux/4 -> Servo_RBF/1(In)
  Demux/5 -> Servo_PBF/1(In)
  Demux1/4 -> Sum3/1
  Demux1/5 -> Sum4/1
  Sum3/1 -> gain_actBFR/1
  Sum4/1 -> gain_actBFP/1
  Servo_YBF/1(Out) -> gainBFY/1, Mux2/6
  Demux/6 -> Servo_YBF/1(In)
  Demux1/6 -> Sum5/1
  gain_actBFV/1 -> Mux1/3
  gain_actBFY/1 -> Mux1/6
  gain_actBFR/1 -> Mux1/4
  gain_actBFT/1 -> Mux1/2
  gain_actBFL/1 -> Mux1/1
  gain_actBFP/1 -> Mux1/5
  BPCOMB/1 -> Demux2/1
  Demux2/2 -> Sum7/1
  Demux2/1 -> Sum6/1
  Demux2/3 -> Sum11/1
  Sum/1 -> Sum6/2
  Sum6/1 -> gain_actBFL/1
  Sum1/1 -> Sum7/2
  Sum7/1 -> gain_actBFT/1
  Sum5/1 -> Sum11/2
  Sum11/1 -> gain_actBFY/1
  gainBFY/1 -> Sum5/2
  gainBFR/1 -> Sum3/2
  gainBFT/1 -> Sum1/2
  gainBFV/1 -> Sum2/2
  gainBFL/1 -> Sum/2
  gainBFP/1 -> Sum4/2

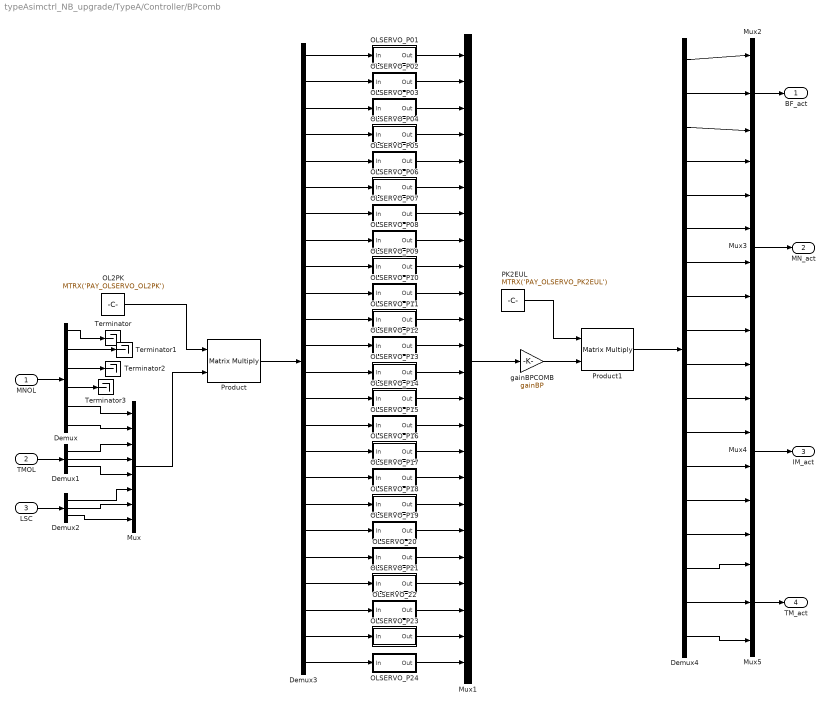
== system typeAsimctrl_NB_upgrade/TypeA/Controller/BPcomb ==
  MNOL : Inport
  TMOL : Inport  Port=2
  LSC : Inport  Port=3
  Demux : Demux  Outputs=6
  Demux1 : Demux  Outputs=3
  Demux2 : Demux  Outputs=3
  Demux3 : Demux  Outputs=24
  Demux4 : Demux  Outputs=18
  Mux : Mux  Inputs=8
  Mux1 : Mux  Inputs=24
  Mux2 : Mux  Inputs=3
  Mux3 : Mux  Inputs=6
  Mux4 : Mux  Inputs=6
  Mux5 : Mux  Inputs=3
  OL2PK : Constant  Value=MTRX('PAY_OLSERVO_OL2PK')
  OLSERVO_20 : Subsystem
  OLSERVO_22 : Subsystem
  OLSERVO_P01 : Subsystem
  OLSERVO_P02 : Subsystem
  OLSERVO_P03 : Subsystem
  OLSERVO_P04 : Subsystem
  OLSERVO_P05 : Subsystem
  OLSERVO_P06 : Subsystem
  OLSERVO_P07 : Subsystem
  OLSERVO_P08 : Subsystem
  OLSERVO_P09 : Subsystem
  OLSERVO_P10 : Subsystem
  OLSERVO_P11 : Subsystem
  OLSERVO_P12 : Subsystem
  OLSERVO_P13 : Subsystem
  OLSERVO_P14 : Subsystem
  OLSERVO_P15 : Subsystem
  OLSERVO_P16 : Subsystem
  OLSERVO_P17 : Subsystem
  OLSERVO_P18 : Subsystem
  OLSERVO_P19 : Subsystem
  OLSERVO_P21 : Subsystem
  OLSERVO_P23 : Subsystem
  OLSERVO_P24 : Subsystem
  PK2EUL : Constant  Value=MTRX('PAY_OLSERVO_PK2EUL')
  Product : Product  Multiplication=Matrix(*)
  Product1 : Product  Multiplication=Matrix(*)
  Terminator{,1..3} (4 alike) : Terminator
  gainBPCOMB : Gain  Gain=gainBP
  BF_act : Outport
  MN_act : Outport  Port=2
  IM_act : Outport  Port=3
  TM_act : Outport  Port=4
  wires:
  OL2PK/1 -> Product/1
  MNOL/1 -> Demux/1
  TMOL/1 -> Demux1/1
  LSC/1 -> Demux2/1
  Demux1/1 -> Mux/3
  Demux1/2 -> Mux/4
  Demux1/3 -> Mux/5
  Demux2/1 -> Mux/6
  Demux2/2 -> Mux/7
  Demux2/3 -> Mux/8
  Mux/1 -> Product/2
  Product/1 -> Demux3/1
  Demux3/1 -> OLSERVO_P01/1(In)
  Demux3/2 -> OLSERVO_P02/1(In)
  Demux3/3 -> OLSERVO_P03/1(In)
  Demux3/4 -> OLSERVO_P04/1(In)
  Demux3/5 -> OLSERVO_P05/1(In)
  Demux3/6 -> OLSERVO_P06/1(In)
  Demux3/7 -> OLSERVO_P07/1(In)
  Demux3/8 -> OLSERVO_P08/1(In)
  Demux3/9 -> OLSERVO_P09/1(In)
  Demux3/10 -> OLSERVO_P10/1(In)
  Demux3/11 -> OLSERVO_P11/1(In)
  Demux3/12 -> OLSERVO_P12/1(In)
  Demux3/13 -> OLSERVO_P13/1(In)
  Demux3/14 -> OLSERVO_P14/1(In)
  Demux3/15 -> OLSERVO_P15/1(In)
  Demux3/16 -> OLSERVO_P16/1(In)
  Demux3/17 -> OLSERVO_P17/1(In)
  Demux3/18 -> OLSERVO_P18/1(In)
  Demux3/19 -> OLSERVO_P19/1(In)
  Demux3/20 -> OLSERVO_20/1(In)
  Demux3/21 -> OLSERVO_P21/1(In)
  Demux3/22 -> OLSERVO_22/1(In)
  Demux3/23 -> OLSERVO_P23/1(In)
  Demux3/24 -> OLSERVO_P24/1(In)
  OLSERVO_P01/1(Out) -> Mux1/1
  OLSERVO_P02/1(Out) -> Mux1/2
  OLSERVO_P03/1(Out) -> Mux1/3
  OLSERVO_P04/1(Out) -> Mux1/4
  OLSERVO_P05/1(Out) -> Mux1/5
  OLSERVO_P06/1(Out) -> Mux1/6
  OLSERVO_P07/1(Out) -> Mux1/7
  OLSERVO_P08/1(Out) -> Mux1/8
  OLSERVO_P09/1(Out) -> Mux1/9
  OLSERVO_P10/1(Out) -> Mux1/10
  OLSERVO_P11/1(Out) -> Mux1/11
  OLSERVO_P12/1(Out) -> Mux1/12
  OLSERVO_P13/1(Out) -> Mux1/13
  OLSERVO_P14/1(Out) -> Mux1/14
  OLSERVO_P15/1(Out) -> Mux1/15
  OLSERVO_P16/1(Out) -> Mux1/16
  OLSERVO_P17/1(Out) -> Mux1/17
  OLSERVO_P18/1(Out) -> Mux1/18
  OLSERVO_P19/1(Out) -> Mux1/19
  OLSERVO_20/1(Out) -> Mux1/20
  OLSERVO_P21/1(Out) -> Mux1/21
  OLSERVO_22/1(Out) -> Mux1/22
  OLSERVO_P23/1(Out) -> Mux1/23
  OLSERVO_P24/1(Out) -> Mux1/24
  Mux1/1 -> gainBPCOMB/1
  PK2EUL/1 -> Product1/1
  Product1/1 -> Demux4/1
  Demux4/1 -> Mux2/1
  Demux4/2 -> Mux2/2
  Demux4/3 -> Mux2/3
  Mux2/1 -> BF_act/1
  Demux4/5 -> Mux3/2
  Demux4/4 -> Mux3/1
  Demux4/6 -> Mux3/3
  Demux4/7 -> Mux3/4
  Demux4/8 -> Mux3/5
  Demux4/9 -> Mux3/6
  Mux3/1 -> MN_act/1
  Demux4/11 -> Mux4/2
  Demux4/10 -> Mux4/1
  Demux4/12 -> Mux4/3
  Demux4/13 -> Mux4/4
  Demux4/14 -> Mux4/5
  Demux4/15 -> Mux4/6
  Mux4/1 -> IM_act/1
  Demux4/16 -> Mux5/1
  Demux4/17 -> Mux5/2
  Demux4/18 -> Mux5/3
  Mux5/1 -> TM_act/1
  Demux/1 -> Terminator/1
  gainBPCOMB/1 -> Product1/2
  Demux/5 -> Mux/1
  Demux/6 -> Mux/2
  Demux/2 -> Terminator1/1
  Demux/3 -> Terminator2/1
  Demux/4 -> Terminator3/1

== system typeAsimctrl_NB_upgrade/TypeA/Controller/GASservo ==
  GAS_LVDT : Inport
  injGAS : Inport  Port=2
  Demux : Demux  Outputs=5
  Demux1 : Demux  Outputs=5
  Mux1 : Mux  Inputs=5
  Mux2 : Mux  Inputs=5
  Servo_GASBF : Subsystem
  Servo_GASF0 : Subsystem
  Servo_GASF1 : Subsystem
  Servo_GASF2 : Subsystem
  Servo_GASF3 : Subsystem
  Sum{,1..4} (5 alike) : Sum  Inputs=++|
  gainGASBF : Gain  Gain=gainGASBF
  gainGASF0 : Gain  Gain=gainGASF0
  gainGASF1 : Gain  Gain=gainGASF1
  gainGASF2 : Gain  Gain=gainGASF2
  gainGASF3 : Gain  Gain=gainGASF3
  gain_actGASBF : Gain  Gain=gain_actBFGAS
  gain_actGASF0 : Gain  Gain=gain_actF0GAS
  gain_actGASF1 : Gain  Gain=gain_actF1GAS
  gain_actGASF2 : Gain  Gain=gain_actF2GAS
  gain_actGASF3 : Gain  Gain=gain_actF3GAS
  actGAS : Outport
  fbGAS : Outport  Port=2
  wires:
  GAS_LVDT/1 -> Demux/1
  Demux/1 -> Servo_GASF0/1(In)
  Demux/2 -> Servo_GASF1/1(In)
  Demux/3 -> Servo_GASF2/1(In)
  Servo_GASF0/1(Out) -> gainGASF0/1, Mux2/1
  Servo_GASF1/1(Out) -> gainGASF1/1, Mux2/2
  Servo_GASF2/1(Out) -> gainGASF2/1, Mux2/3
  injGAS/1 -> Demux1/1
  Mux1/1 -> actGAS/1
  Mux2/1 -> fbGAS/1
  Demux1/3 -> Sum2/1
  Demux1/2 -> Sum1/1
  Demux1/1 -> Sum/1
  Servo_GASF3/1(Out) -> gainGASF3/1, Mux2/4
  Servo_GASBF/1(Out) -> gainGASBF/1, Mux2/5
  Demux/4 -> Servo_GASF3/1(In)
  Demux/5 -> Servo_GASBF/1(In)
  Demux1/4 -> Sum3/1
  Demux1/5 -> Sum4/1
  gain_actGASF0/1 -> Mux1/1
  gain_actGASF2/1 -> Mux1/3
  gain_actGASF1/1 -> Mux1/2
  gain_actGASF3/1 -> Mux1/4
  gain_actGASBF/1 -> Mux1/5
  Sum/1 -> gain_actGASF0/1
  Sum2/1 -> gain_actGASF2/1
  Sum1/1 -> gain_actGASF1/1
  Sum3/1 -> gain_actGASF3/1
  Sum4/1 -> gain_actGASBF/1
  gainGASBF/1 -> Sum4/2
  gainGASF1/1 -> Sum1/2
  gainGASF2/1 -> Sum2/2
  gainGASF3/1 -> Sum3/2
  gainGASF0/1 -> Sum/2

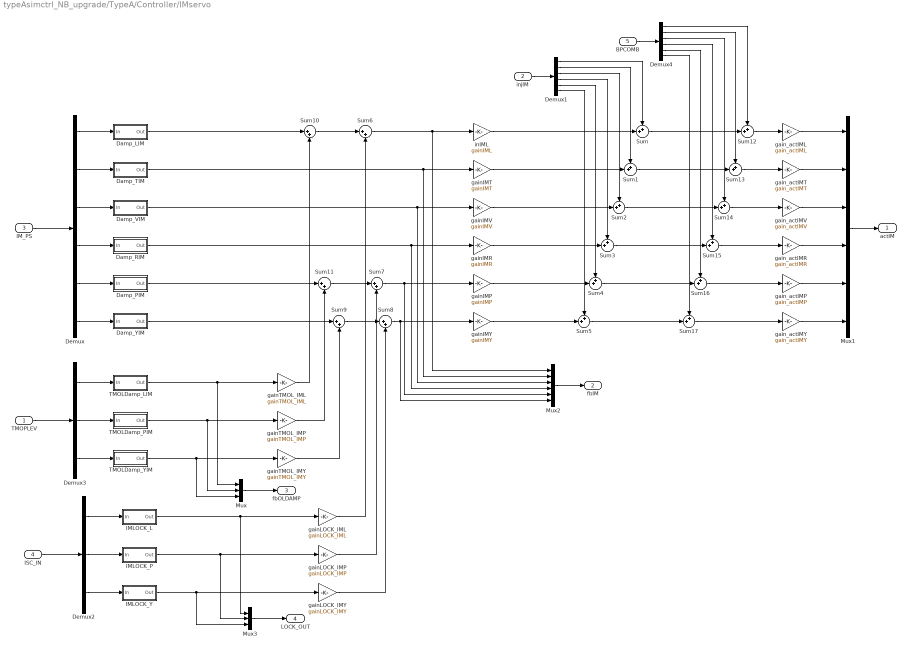
== system typeAsimctrl_NB_upgrade/TypeA/Controller/IMservo ==
  TMOPLEV : Inport
  injIM : Inport  Port=2
  IM_PS : Inport  Port=3
  ISC_IN : Inport  Port=4
  BPCOMB : Inport  Port=5
  Damp_LIM : Subsystem
  Damp_PIM : Subsystem
  Damp_RIM : Subsystem
  Damp_TIM : Subsystem
  Damp_VIM : Subsystem
  Damp_YIM : Subsystem
  Demux : Demux  Outputs=6
  Demux1 : Demux  Outputs=6
  Demux2 : Demux  Outputs=3
  Demux3 : Demux  Outputs=3
  Demux4 : Demux  Outputs=6
  IMLOCK_L : Subsystem
  IMLOCK_P : Subsystem
  IMLOCK_Y : Subsystem
  Mux : Mux  Inputs=3
  Mux1 : Mux  Inputs=6
  Mux2 : Mux  Inputs=6
  Mux3 : Mux  Inputs=3
  Sum{,1..5,12..17} (12 alike) : Sum  Inputs=++|
  Sum{6..11} (6 alike) : Sum  Inputs=|++
  TMOLDamp_LIM : Subsystem
  TMOLDamp_PIM : Subsystem
  TMOLDamp_YIM : Subsystem
  gainIMP : Gain  Gain=gainIMP
  gainIMR : Gain  Gain=gainIMR
  gainIMT : Gain  Gain=gainIMT
  gainIMV : Gain  Gain=gainIMV
  gainIMY : Gain  Gain=gainIMY
  gainLOCK_IML : Gain  Gain=gainLOCK_IML
  gainLOCK_IMP : Gain  Gain=gainLOCK_IMP
  gainLOCK_IMY : Gain  Gain=gainLOCK_IMY
  gainTMOL_IML : Gain  Gain=gainTMOL_IML
  gainTMOL_IMP : Gain  Gain=gainTMOL_IMP
  gainTMOL_IMY : Gain  Gain=gainTMOL_IMY
  gain_actIML : Gain  Gain=gain_actIML
  gain_actIMP : Gain  Gain=gain_actIMP
  gain_actIMR : Gain  Gain=gain_actIMR
  gain_actIMT : Gain  Gain=gain_actIMT
  gain_actIMV : Gain  Gain=gain_actIMV
  gain_actIMY : Gain  Gain=gain_actIMY
  inIML : Gain  Gain=gainIML
  actIM : Outport
  fbIM : Outport  Port=2
  fbOLDAMP : Outport  Port=3
  LOCK_OUT : Outport  Port=4
  wires:
  injIM/1 -> Demux1/1
  Mux1/1 -> actIM/1
  Mux2/1 -> fbIM/1
  Demux1/3 -> Sum2/1
  Demux1/2 -> Sum1/1
  Demux1/1 -> Sum/1
  Demux1/4 -> Sum3/1
  Demux1/5 -> Sum4/1
  Demux1/6 -> Sum5/1
  gain_actIMV/1 -> Mux1/3
  gain_actIMY/1 -> Mux1/6
  gain_actIMR/1 -> Mux1/4
  gain_actIMT/1 -> Mux1/2
  gain_actIML/1 -> Mux1/1
  gain_actIMP/1 -> Mux1/5
  TMOPLEV/1 -> Demux3/1
  Demux3/1 -> TMOLDamp_LIM/1(In)
  Demux3/2 -> TMOLDamp_PIM/1(In)
  Demux3/3 -> TMOLDamp_YIM/1(In)
  TMOLDamp_LIM/1(Out) -> Mux/1, gainTMOL_IML/1
  TMOLDamp_PIM/1(Out) -> Mux/2, gainTMOL_IMP/1
  TMOLDamp_YIM/1(Out) -> Mux/3, gainTMOL_IMY/1
  IM_PS/1 -> Demux/1
  Demux/1 -> Damp_LIM/1(In)
  Demux/2 -> Damp_TIM/1(In)
  Demux/3 -> Damp_VIM/1(In)
  Demux/4 -> Damp_RIM/1(In)
  Demux/5 -> Damp_PIM/1(In)
  Demux/6 -> Damp_YIM/1(In)
  Damp_LIM/1(Out) -> Sum10/1
  Damp_TIM/1(Out) -> Mux2/2, gainIMT/1
  Damp_VIM/1(Out) -> Mux2/3, gainIMV/1
  Damp_RIM/1(Out) -> Mux2/4, gainIMR/1
  Damp_PIM/1(Out) -> Sum11/1
  Damp_YIM/1(Out) -> Sum9/1
  Mux/1 -> fbOLDAMP/1
  ISC_IN/1 -> Demux2/1
  Demux2/1 -> IMLOCK_L/1(In)
  Demux2/2 -> IMLOCK_P/1(In)
  Demux2/3 -> IMLOCK_Y/1(In)
  IMLOCK_L/1(Out) -> gainLOCK_IML/1, Mux3/1
  IMLOCK_P/1(Out) -> gainLOCK_IMP/1, Mux3/2
  IMLOCK_Y/1(Out) -> gainLOCK_IMY/1, Mux3/3
  Mux3/1 -> LOCK_OUT/1
  Sum10/1 -> Sum6/1
  Sum6/1 -> Mux2/1, inIML/1
  Sum9/1 -> Sum8/1
  Sum8/1 -> Mux2/6, gainIMY/1
  Sum11/1 -> Sum7/1
  Sum7/1 -> Mux2/5, gainIMP/1
  BPCOMB/1 -> Demux4/1
  Demux4/3 -> Sum14/1
  Demux4/2 -> Sum13/1
  Demux4/1 -> Sum12/1
  Demux4/4 -> Sum15/1
  Demux4/5 -> Sum16/1
  Demux4/6 -> Sum17/1
  Sum/1 -> Sum12/2
  Sum12/1 -> gain_actIML/1
  Sum1/1 -> Sum13/2
  Sum13/1 -> gain_actIMT/1
  Sum2/1 -> Sum14/2
  Sum14/1 -> gain_actIMV/1
  Sum3/1 -> Sum15/2
  Sum15/1 -> gain_actIMR/1
  Sum4/1 -> Sum16/2
  Sum16/1 -> gain_actIMP/1
  Sum5/1 -> Sum17/2
  Sum17/1 -> gain_actIMY/1
  gainLOCK_IML/1 -> Sum6/2
  gainLOCK_IMY/1 -> Sum8/2
  gainLOCK_IMP/1 -> Sum7/2
  gainTMOL_IMY/1 -> Sum9/2
  gainTMOL_IMP/1 -> Sum11/2
  gainTMOL_IML/1 -> Sum10/2
  gainIMV/1 -> Sum2/2
  gainIMR/1 -> Sum3/2
  gainIMY/1 -> Sum5/2
  inIML/1 -> Sum/2
  gainIMT/1 -> Sum1/2
  gainIMP/1 -> Sum4/2

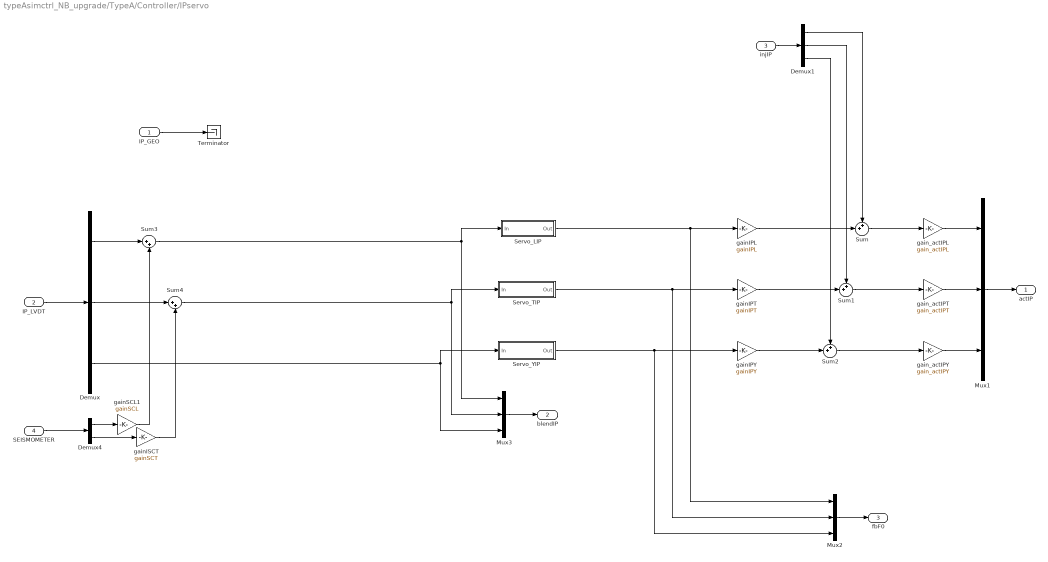
== system typeAsimctrl_NB_upgrade/TypeA/Controller/IPservo ==
  IP_GEO : Inport
  IP_LVDT : Inport  Port=2
  injIP : Inport  Port=3
  SEISMOMETER : Inport  Port=4
  Demux : Demux  Outputs=3
  Demux1 : Demux  Outputs=3
  Demux4 : Demux  Outputs=2
  Mux1 : Mux  Inputs=3
  Mux2 : Mux  Inputs=3
  Mux3 : Mux  Inputs=3
  Servo_LIP : Subsystem
  Servo_TIP : Subsystem
  Servo_YIP : Subsystem
  Sum : Sum  Inputs=++|
  Sum1 : Sum  Inputs=++|
  Sum2 : Sum  Inputs=++|
  Sum3 : Sum  Inputs=|++
  Sum4 : Sum  Inputs=|++
  Terminator : Terminator
  gainIPL : Gain  Gain=gainIPL
  gainIPT : Gain  Gain=gainIPT
  gainIPY : Gain  Gain=gainIPY
  gainISCT : Gain  Gain=gainSCT
  gainSCL1 : Gain  Gain=gainSCL
  gain_actIPL : Gain  Gain=gain_actIPL
  gain_actIPT : Gain  Gain=gain_actIPT
  gain_actIPY : Gain  Gain=gain_actIPY
  actIP : Outport
  blendIP : Outport  Port=2
  fbF0 : Outport  Port=3
  wires:
  IP_LVDT/1 -> Demux/1
  Servo_LIP/1(Out) -> Mux2/1, gainIPL/1
  Servo_TIP/1(Out) -> Mux2/2, gainIPT/1
  Servo_YIP/1(Out) -> Mux2/3, gainIPY/1
  injIP/1 -> Demux1/1
  Sum1/1 -> gain_actIPT/1
  Sum2/1 -> gain_actIPY/1
  Sum/1 -> gain_actIPL/1
  Mux1/1 -> actIP/1
  Mux2/1 -> fbF0/1
  Demux1/3 -> Sum2/1
  Demux1/2 -> Sum1/1
  Demux1/1 -> Sum/1
  gain_actIPT/1 -> Mux1/2
  gain_actIPL/1 -> Mux1/1
  gain_actIPY/1 -> Mux1/3
  IP_GEO/1 -> Terminator/1
  Sum3/1 -> Servo_LIP/1(In), Mux3/1
  Sum4/1 -> Servo_TIP/1(In), Mux3/2
  Demux/3 -> Servo_YIP/1(In), Mux3/3
  Mux3/1 -> blendIP/1
  SEISMOMETER/1 -> Demux4/1
  Demux/1 -> Sum3/1
  Demux/2 -> Sum4/1
  Demux4/1 -> gainSCL1/1
  Demux4/2 -> gainISCT/1
  gainIPL/1 -> Sum/2
  gainIPT/1 -> Sum1/2
  gainIPY/1 -> Sum2/2
  gainSCL1/1 -> Sum3/2
  gainISCT/1 -> Sum4/2

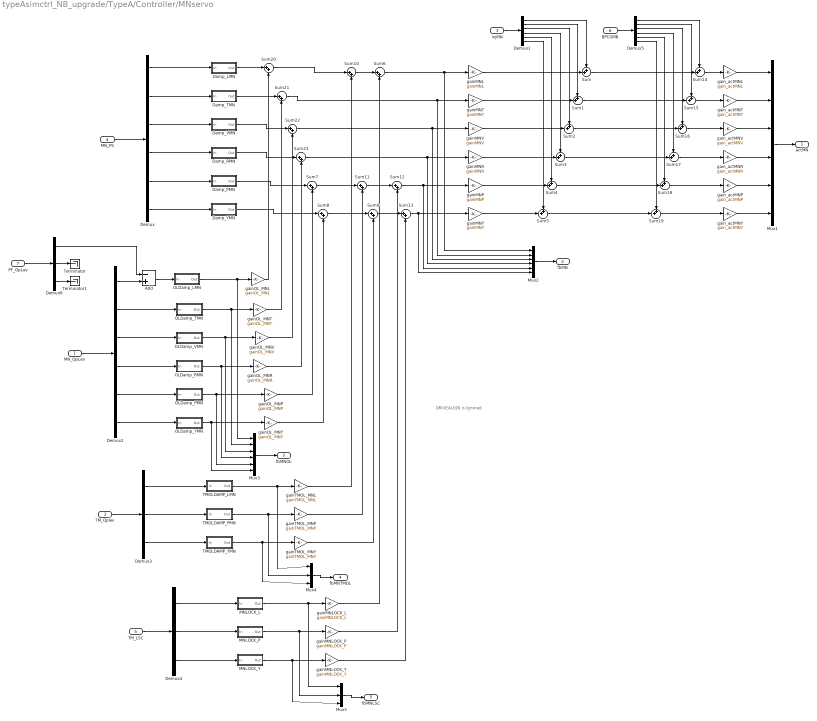
== system typeAsimctrl_NB_upgrade/TypeA/Controller/MNservo ==
  note: DRIVEALIGN is Ignored
  MN_OpLev : Inport
  TM_Oplev : Inport  Port=2
  injMN : Inport  Port=3
  MN_PS : Inport  Port=4
  TM_LSC : Inport  Port=5
  BPCOMB : Inport  Port=6
  PF_OpLev : Inport  Port=7
  Add : Sum  Inputs=-+
  Damp_LMN : Subsystem
  Damp_PMN : Subsystem
  Damp_RMN : Subsystem
  Damp_TMN : Subsystem
  Damp_VMN : Subsystem
  Damp_YMN : Subsystem
  Demux{,1..2,5} (4 alike) : Demux  Outputs=6
  Demux3 : Demux  Outputs=3
  Demux4 : Demux  Outputs=3
  Demux6 : Demux  Outputs=3
  MNLOCK_L : Subsystem
  MNLOCK_P : Subsystem
  MNLOCK_Y : Subsystem
  Mux1 : Mux  Inputs=6
  Mux2 : Mux  Inputs=6
  Mux3 : Mux  Inputs=6
  Mux4 : Mux  Inputs=3
  Mux5 : Mux  Inputs=3
  OLDamp_LMN : Subsystem
  OLDamp_PMN : Subsystem
  OLDamp_RMN : Subsystem
  OLDamp_TMN : Subsystem
  OLDamp_VMN : Subsystem
  OLDamp_YMN : Subsystem
  Sum{,1..5,14..19} (12 alike) : Sum  Inputs=++|
  Sum{6..13,20..23} (12 alike) : Sum  Inputs=|++
  TMOLDAMP_LMN : Subsystem
  TMOLDAMP_PMN : Subsystem
  TMOLDAMP_YMN : Subsystem
  Terminator : Terminator
  Terminator1 : Terminator
  gainMNL : Gain  Gain=gainMNL
  gainMNLOCK_L : Gain  Gain=gainMNLOCK_L
  gainMNLOCK_P : Gain  Gain=gainMNLOCK_P
  gainMNLOCK_Y : Gain  Gain=gainMNLOCK_Y
  gainMNP : Gain  Gain=gainMNP
  gainMNR : Gain  Gain=gainMNR
  gainMNT : Gain  Gain=gainMNT
  gainMNV : Gain  Gain=gainMNV
  gainMNY : Gain  Gain=gainMNY
  gainOL_MNL : Gain  Gain=gainOL_MNL
  gainOL_MNP : Gain  Gain=gainOL_MNP
  gainOL_MNR : Gain  Gain=gainOL_MNR
  gainOL_MNT : Gain  Gain=gainOL_MNT
  gainOL_MNV : Gain  Gain=gainOL_MNV
  gainOL_MNY : Gain  Gain=gainOL_MNY
  gainTMOL_MNL : Gain  Gain=gainTMOL_MNL
  gainTMOL_MNP : Gain  Gain=gainTMOL_MNP
  gainTMOL_MNY : Gain  Gain=gainTMOL_MNY
  gain_actMNL : Gain  Gain=gain_actMNL
  gain_actMNP : Gain  Gain=gain_actMNP
  gain_actMNR : Gain  Gain=gain_actMNR
  gain_actMNT : Gain  Gain=gain_actMNT
  gain_actMNV : Gain  Gain=gain_actMNV
  gain_actMNY : Gain  Gain=gain_actMNY
  actMN : Outport
  fbMN : Outport  Port=2
  fbMNOL : Outport  Port=3
  fbMNTMOL : Outport  Port=4
  fbMNLSC : Outport  Port=5
  wires:
  injMN/1 -> Demux1/1
  Mux1/1 -> actMN/1
  Mux2/1 -> fbMN/1
  Demux1/3 -> Sum2/1
  Demux1/2 -> Sum1/1
  Demux1/1 -> Sum/1
  Demux1/4 -> Sum3/1
  Demux1/5 -> Sum4/1
  Demux1/6 -> Sum5/1
  gain_actMNV/1 -> Mux1/3
  gain_actMNY/1 -> Mux1/6
  gain_actMNR/1 -> Mux1/4
  gain_actMNT/1 -> Mux1/2
  gain_actMNL/1 -> Mux1/1
  gain_actMNP/1 -> Mux1/5
  TMOLDAMP_YMN/1(Out) -> Mux4/3, gainTMOL_MNY/1
  OLDamp_PMN/1(Out) -> Mux3/5, gainOL_MNP/1
  OLDamp_YMN/1(Out) -> Mux3/6, gainOL_MNY/1
  MN_OpLev/1 -> Demux2/1
  TM_Oplev/1 -> Demux3/1
  Demux3/1 -> TMOLDAMP_LMN/1(In)
  gainOL_MNP/1 -> Sum7/2
  gainOL_MNY/1 -> Sum8/2
  Sum7/1 -> Sum11/1
  gainTMOL_MNL/1 -> Sum10/2
  gainTMOL_MNP/1 -> Sum11/2
  gainTMOL_MNY/1 -> Sum9/2
  Sum8/1 -> Sum9/1
  Demux3/2 -> TMOLDAMP_PMN/1(In)
  Demux3/3 -> TMOLDAMP_YMN/1(In)
  Sum21/1 -> Mux2/2, gainMNT/1
  Sum22/1 -> Mux2/3, gainMNV/1
  Sum23/1 -> Mux2/4, gainMNR/1
  MN_PS/1 -> Demux/1
  Demux/1 -> Damp_LMN/1(In)
  Demux/2 -> Damp_TMN/1(In)
  Demux/3 -> Damp_VMN/1(In)
  Demux/4 -> Damp_RMN/1(In)
  Demux/5 -> Damp_PMN/1(In)
  Demux/6 -> Damp_YMN/1(In)
  Damp_PMN/1(Out) -> Sum7/1
  Damp_YMN/1(Out) -> Sum8/1
  TM_LSC/1 -> Demux4/1
  Demux4/1 -> MNLOCK_L/1(In)
  gainMNLOCK_L/1 -> Sum6/2
  gainMNLOCK_P/1 -> Sum12/2
  gainMNLOCK_Y/1 -> Sum13/2
  Demux4/2 -> MNLOCK_P/1(In)
  Demux4/3 -> MNLOCK_Y/1(In)
  Sum10/1 -> Sum6/1
  Sum6/1 -> Mux2/1, gainMNL/1
  Sum12/1 -> Mux2/5, gainMNP/1
  Sum11/1 -> Sum12/1
  Sum9/1 -> Sum13/1
  Sum13/1 -> Mux2/6, gainMNY/1
  BPCOMB/1 -> Demux5/1
  Demux5/3 -> Sum16/1
  Demux5/2 -> Sum15/1
  Demux5/1 -> Sum14/1
  Demux5/4 -> Sum17/1
  Demux5/5 -> Sum18/1
  Demux5/6 -> Sum19/1
  Sum/1 -> Sum14/2
  Sum14/1 -> gain_actMNL/1
  Sum1/1 -> Sum15/2
  Sum15/1 -> gain_actMNT/1
  Sum2/1 -> Sum16/2
  Sum16/1 -> gain_actMNV/1
  Sum3/1 -> Sum17/2
  Sum17/1 -> gain_actMNR/1
  Sum4/1 -> Sum18/2
  Sum18/1 -> gain_actMNP/1
  Sum5/1 -> Sum19/2
  Sum19/1 -> gain_actMNY/1
  gainMNL/1 -> Sum/2
  gainMNR/1 -> Sum3/2
  gainMNP/1 -> Sum4/2
  gainMNT/1 -> Sum1/2
  gainMNY/1 -> Sum5/2
  gainMNV/1 -> Sum2/2
  Mux3/1 -> fbMNOL/1
  TMOLDAMP_PMN/1(Out) -> Mux4/2, gainTMOL_MNP/1
  Mux4/1 -> fbMNTMOL/1
  TMOLDAMP_LMN/1(Out) -> Mux4/1, gainTMOL_MNL/1
  MNLOCK_Y/1(Out) -> Mux5/3, gainMNLOCK_Y/1
  MNLOCK_P/1(Out) -> Mux5/2, gainMNLOCK_P/1
  Mux5/1 -> fbMNLSC/1
  MNLOCK_L/1(Out) -> Mux5/1, gainMNLOCK_L/1
  Demux2/5 -> OLDamp_PMN/1(In)
  Demux2/6 -> OLDamp_YMN/1(In)
  PF_OpLev/1 -> Demux6/1
  Demux6/2 -> Terminator/1
  Demux6/3 -> Terminator1/1
  Demux6/1 -> Add/1
  Demux2/1 -> Add/2
  Add/1 -> OLDamp_LMN/1(In)
  OLDamp_RMN/1(Out) -> Mux3/4, gainOL_MNR/1
  OLDamp_VMN/1(Out) -> Mux3/3, gainOL_MNV/1
  OLDamp_TMN/1(Out) -> Mux3/2, gainOL_MNT/1
  OLDamp_LMN/1(Out) -> Mux3/1, gainOL_MNL/1
  Demux2/2 -> OLDamp_TMN/1(In)
  Demux2/3 -> OLDamp_VMN/1(In)
  Demux2/4 -> OLDamp_RMN/1(In)
  Damp_LMN/1(Out) -> Sum20/1
  Sum20/1 -> Sum10/1
  Damp_TMN/1(Out) -> Sum21/1
  Damp_VMN/1(Out) -> Sum22/1
  Damp_RMN/1(Out) -> Sum23/1
  gainOL_MNR/1 -> Sum23/2
  gainOL_MNV/1 -> Sum22/2
  gainOL_MNT/1 -> Sum21/2
  gainOL_MNL/1 -> Sum20/2
